simulink model "Robust_joint_Space"  (R2020b)
settings: Solver=VariableStepAuto  StartTime=0.0  StopTime=10  RelTol=1e-3
(part 7 of 7)

== matlab function Robust_joint_Space/robust inverse dynamic controller/M_hat_prod ==
  data: m input; Mhat output; theta input
function Mhat = Find_M(m,theta)

m1 = m(1);
m2 = m(2);
m3 = m(3);
m4 = m(4);
m5 = m(5);
m6 = m(6);

t1 = theta(1);
t2 = theta(2);
t3 = theta(3);
t4 = theta(4);
t5 = theta(5);
t6 = theta(6);

L1=0.1025;
L2=0.408;
L3=0.376;
L4=0.1025; 
L5=0.1025;

Mhat =[(78961*m2)/4 + (411889*m3)/4 + (694641*m4)/4 + (1431307*m5)/8 + (1431307*m6)/8 + (61463515545781917*cos(2*t2))/1152921504606846976 - 83232*m3*cos(2*t2) - 83232*m4*cos(2*t2) - 83232*m5*cos(2*t2) - 83232*m6*cos(2*t2) - (42025*m5*cos(2*t2 + 2*t3 + 2*t4))/8 - (42025*m6*cos(2*t2 + 2*t3 + 2*t4))/8 - 281*L1*m3 - 281*L1*m4 - (205*L4*m5)/2 - 70688*m4*cos(2*t2 + 2*t3) - 70688*m5*cos(2*t2 + 2*t3) - 70688*m6*cos(2*t2 + 2*t3) - 41820*m5*cos(2*t2 + t3 + t4) - 41820*m6*cos(2*t2 + t3 + t4) + 41820*m5*cos(t3 + t4) + 41820*m6*cos(t3 + t4) + L1^2*m3 + (L2^2*m2)/8 + L1^2*m4 + (3*L3^2*m5)/16 + (L4^2*m5)/2 + 153408*m4*cos(t3) + 153408*m5*cos(t3) + 38540*m5*cos(t4) + 153408*m6*cos(t3) + 38540*m6*cos(t4) - 38540*m5*cos(2*t2 + 2*t3 + t4) - 38540*m6*cos(2*t2 + 2*t3 + t4) - 153408*m4*cos(2*t2 + t3) - 153408*m5*cos(2*t2 + t3) - 153408*m6*cos(2*t2 + t3) + 102*L3*m5*cos(2*t2 + t3 + t4 + t5) + 94*L3*m5*cos(t4 - t5) - (205*L3*m5*cos(2*t2 + 2*t3 + 2*t4 - t5))/8 - 102*L3*m5*cos(t3 + t4 + t5) + (205*L4*m5*cos(2*t2 + 2*t3 + 2*t4))/2 - 102*L3*m5*cos(2*t2 + t3 + t4 - t5) + 94*L3*m5*cos(2*t2 + 2*t3 + t4 + t5) - (L3^2*m5*cos(2*t2 + 2*t3 + 2*t4 - 2*t5))/32 - (L3^2*m5*cos(2*t2 + 2*t3 + 2*t4 + 2*t5))/32 + 408*L4*m5*cos(2*t2 + t3 + t4) + 102*L3*m5*cos(t3 + t4 - t5) - (L2^2*m2*cos(2*t2))/8 + (L3^2*m5*cos(2*t5))/16 + (L3^2*m5*cos(2*t2 + 2*t3 + 2*t4))/16 - (L4^2*m5*cos(2*t2 + 2*t3 + 2*t4))/2 - 408*L4*m5*cos(t3 + t4) - 94*L3*m5*cos(t4 + t5) - 94*L3*m5*cos(2*t2 + 2*t3 + t4 - t5) + (205*L3*m5*cos(2*t2 + 2*t3 + 2*t4 + t5))/8 + (281*L3*m5*cos(t5))/2 - 376*L4*m5*cos(t4) + 376*L4*m5*cos(2*t2 + 2*t3 + t4) - (L3*L4*m5*cos(2*t2 + 2*t3 + 2*t4 + t5))/4 + (L3*L4*m5*cos(2*t2 + 2*t3 + 2*t4 - t5))/4 + 204764811175443545/1152921504606846976,                                                                                                                                                                      (61463515545781917*cos(t1 + 2*t2))/2305843009213693952 - (61463515545781917*cos(t1 - 2*t2))/2305843009213693952 - 52828*m4*cos(t2 + t3) - 52828*m5*cos(t2 + t3) - 52828*m6*cos(t2 + t3) - 57324*m3*cos(t2) - 57324*m4*cos(t2) - 57324*m5*cos(t2) - 57324*m6*cos(t2) - (57605*m5*cos(t2 + t3 + t4))/4 - (57605*m6*cos(t2 + t3 + t4))/4 - (243*L3*m5*cos(t2 + t3 + t4 - t5))/4 - (281*L2*m2*cos(t1 - t2))/8 - 102*L3*m5*cos(t2 - t5) - 94*L3*m5*cos(t2 + t3 + t5) + (281*L4*m5*cos(t2 + t3 + t4))/2 - (L3^2*m5*cos(t2 + t3 + t4 - 2*t5))/16 + (L3^2*m5*cos(t2 + t3 + t4 + 2*t5))/16 - (L2^2*m2*cos(t1 - 2*t2))/16 + (L2^2*m2*cos(t1 + 2*t2))/16 - 94*L3*m5*cos(t2 + t3 - t5) + (19*L3*m5*cos(t2 + t3 + t4 + t5))/2 - (281*L2*m2*cos(t1 + t2))/8 + 376*L1*m4*cos(t2 + t3) - 102*L3*m5*cos(t2 + t5) + 408*L1*m3*cos(t2) + 408*L1*m4*cos(t2) + (L3*L4*m5*cos(t2 + t3 + t4 - t5))/4 + (L3*L4*m5*cos(t2 + t3 + t4 + t5))/4,                                                                                                                                                                                                                                                                                                      (1690603261718859*cos(t1 - 2*t2))/2305843009213693952 - (1690603261718859*cos(t1 + 2*t2))/2305843009213693952 - 52828*m4*cos(t2 + t3) - 52828*m5*cos(t2 + t3) - 52828*m6*cos(t2 + t3) - (57605*m5*cos(t2 + t3 + t4))/4 - (57605*m6*cos(t2 + t3 + t4))/4 - (243*L3*m5*cos(t2 + t3 + t4 - t5))/4 - 94*L3*m5*cos(t2 + t3 + t5) + (281*L4*m5*cos(t2 + t3 + t4))/2 - (L3^2*m5*cos(t2 + t3 + t4 - 2*t5))/16 + (L3^2*m5*cos(t2 + t3 + t4 + 2*t5))/16 - 94*L3*m5*cos(t2 + t3 - t5) + (19*L3*m5*cos(t2 + t3 + t4 + t5))/2 + 376*L1*m4*cos(t2 + t3) + (L3*L4*m5*cos(t2 + t3 + t4 - t5))/4 + (L3*L4*m5*cos(t2 + t3 + t4 + t5))/4,                                                                                                                                                                                                                                                                                                                                                                                                                 (1690603261718859*cos(t1 - 2*t2))/2305843009213693952 - (1690603261718859*cos(t1 + 2*t2))/2305843009213693952 - (57605*m5*cos(t2 + t3 + t4))/4 - (57605*m6*cos(t2 + t3 + t4))/4 - (243*L3*m5*cos(t2 + t3 + t4 - t5))/4 + (281*L4*m5*cos(t2 + t3 + t4))/2 - (L3^2*m5*cos(t2 + t3 + t4 - 2*t5))/16 + (L3^2*m5*cos(t2 + t3 + t4 + 2*t5))/16 + (19*L3*m5*cos(t2 + t3 + t4 + t5))/2 + (L3*L4*m5*cos(t2 + t3 + t4 - t5))/4 + (L3*L4*m5*cos(t2 + t3 + t4 + t5))/4,                                                                                                                                                                                                                                                                                                                                                                                                                                                                                                                                                                                                                                             (1690603261718859*cos(t2 + t3 + t4))/1152921504606846976 - (1690603261718859*cos(t1 + t2 - t3 - t4))/4611686018427387904 + (1690603261718859*cos(3*t2 - t1 + t3 + t4))/4611686018427387904 - (1690603261718859*cos(t3 - t2 + t4))/2305843009213693952 - (1690603261718859*cos(3*t2 + t3 + t4))/2305843009213693952 - (1690603261718859*cos(t1 - t2 + t3 + t4))/4611686018427387904 + (1690603261718859*cos(t1 + 3*t2 + t3 + t4))/4611686018427387904 + (19*L3*m5*cos(t2 + t3 + t4 - t5))/2 - 102*L3*m5*cos(t2 - t5) + 94*L3*m5*cos(t2 + t3 + t5) - 94*L3*m5*cos(t2 + t3 - t5) + (L3^2*m5*cos(t2 + t3 + t4))/4 + (243*L3*m5*cos(t2 + t3 + t4 + t5))/4 + 102*L3*m5*cos(t2 + t5) + (L3*L4*m5*cos(t2 + t3 + t4 - t5))/4 - (L3*L4*m5*cos(t2 + t3 + t4 + t5))/4,                                                                                                                                                                                                                                                                                                                                                                                                                                                                                                                                                                                                                                                                                                                                                                                                                                                                                                                                                                                                                                                                                                                                                                               0
                                                                                                                                                                                                                                                                                                                                                                                                                                                                                                                                                                                                                                                                                                                                                                                                                                                          (61463515545781917*cos(t1 + 2*t2))/2305843009213693952 - (61463515545781917*cos(t1 - 2*t2))/2305843009213693952 - 52828*m4*cos(t2 + t3) - 52828*m5*cos(t2 + t3) - 52828*m6*cos(t2 + t3) - 57324*m3*cos(t2) - 57324*m4*cos(t2) - 57324*m5*cos(t2) - 57324*m6*cos(t2) - (57605*m5*cos(t2 + t3 + t4))/4 - (57605*m6*cos(t2 + t3 + t4))/4 - (243*L3*m5*cos(t2 + t3 + t4 - t5))/4 - (281*L2*m2*cos(t1 - t2))/8 - 102*L3*m5*cos(t2 - t5) - 94*L3*m5*cos(t2 + t3 + t5) + (281*L4*m5*cos(t2 + t3 + t4))/2 - (L3^2*m5*cos(t2 + t3 + t4 - 2*t5))/16 + (L3^2*m5*cos(t2 + t3 + t4 + 2*t5))/16 - (L2^2*m2*cos(t1 - 2*t2))/16 + (L2^2*m2*cos(t1 + 2*t2))/16 - 94*L3*m5*cos(t2 + t3 - t5) + (19*L3*m5*cos(t2 + t3 + t4 + t5))/2 - (281*L2*m2*cos(t1 + t2))/8 + 376*L1*m4*cos(t2 + t3) - 102*L3*m5*cos(t2 + t5) + 408*L1*m3*cos(t2) + 408*L1*m4*cos(t2) + (L3*L4*m5*cos(t2 + t3 + t4 - t5))/4 + (L3*L4*m5*cos(t2 + t3 + t4 + t5))/4, (78961*m2)/4 + 166464*m3 + 307840*m4 + (1273385*m5)/4 + (1273385*m6)/4 - (78961*m2*cos(t1)^2)/4 - 205*L4*m5 - (482729437821091191*cos(t1)^2)/4611686018427387904 - (61463515545781917*cos(t2)^2)/576460752303423488 + (1690603261718859*cos(t3)^2)/576460752303423488 + (L3^2*m5)/4 + L4^2*m5 + 306816*m4*cos(t3) + 306816*m5*cos(t3) + 77080*m5*cos(t4) + 306816*m6*cos(t3) + 77080*m6*cos(t4) + (61463515545781917*cos(t1)^2*cos(t2)^2)/576460752303423488 - (1690603261718859*cos(t1)^2*cos(t3)^2)/288230376151711744 + 83640*m5*cos(t3)*cos(t4) + 83640*m6*cos(t3)*cos(t4) - 83640*m5*sin(t3)*sin(t4) - 83640*m6*sin(t3)*sin(t4) + (L2^2*m2*cos(t1)^2)/4 + (L2^2*m2*cos(t2)^2)/4 - (L3^2*m5*cos(t5)^2)/4 - 752*L4*m5*cos(t4) - 816*L4*m5*cos(t3)*cos(t4) - (1690603261718859*cos(t1)*cos(t3)*sin(t1)*sin(t3))/288230376151711744 - (L2^2*m2*cos(t1)^2*cos(t2)^2)/4 + 816*L4*m5*sin(t3)*sin(t4) + 376*L3*m5*sin(t4)*sin(t5) - (281*L2*m2*cos(t1)*sin(t1)*sin(t2))/2 + 408*L3*m5*cos(t3)*sin(t4)*sin(t5) + 408*L3*m5*cos(t4)*sin(t3)*sin(t5) + 1045114580761903793/4611686018427387904,                                                                                                                                                                             141376*m4 + (607529*m5)/4 + (607529*m6)/4 + (2216273498288709*cos(2*t1))/9223372036854775808 + (1690603261718859*cos(2*t2))/2305843009213693952 - (1690603261718859*cos(2*t1 - 2*t2))/4611686018427387904 - (1690603261718859*cos(2*t1 + 2*t2))/4611686018427387904 - (1690603261718859*cos(2*t1 - 2*t3))/1152921504606846976 - 205*L4*m5 + 41820*m5*cos(t3 + t4) + 41820*m6*cos(t3 + t4) + (L3^2*m5)/8 + L4^2*m5 + 153408*m4*cos(t3) + 153408*m5*cos(t3) + 77080*m5*cos(t4) + 153408*m6*cos(t3) + 77080*m6*cos(t4) + 188*L3*m5*cos(t4 - t5) - 102*L3*m5*cos(t3 + t4 + t5) + 102*L3*m5*cos(t3 + t4 - t5) - (L3^2*m5*cos(2*t5))/8 - 408*L4*m5*cos(t3 + t4) - 188*L3*m5*cos(t4 + t5) - 752*L4*m5*cos(t4) + 98563285369573207/9223372036854775808,                                                                                                                                                                                                        (42025*m5)/4 + (42025*m6)/4 + (10637310166265011*cos(2*t1))/9223372036854775808 + (1690603261718859*cos(2*t2))/2305843009213693952 - (1690603261718859*cos(2*t1 - 2*t2))/4611686018427387904 - (1690603261718859*cos(2*t1 + 2*t2))/4611686018427387904 - (1690603261718859*cos(2*t1 - 2*t3))/1152921504606846976 - 205*L4*m5 + 41820*m5*cos(t3 + t4) + 41820*m6*cos(t3 + t4) + (L3^2*m5)/8 + L4^2*m5 + 38540*m5*cos(t4) + 38540*m6*cos(t4) + 94*L3*m5*cos(t4 - t5) - 102*L3*m5*cos(t3 + t4 + t5) + 102*L3*m5*cos(t3 + t4 - t5) - (L3^2*m5*cos(2*t5))/8 - 408*L4*m5*cos(t3 + t4) - 94*L3*m5*cos(t4 + t5) - 376*L4*m5*cos(t4) + 90142248701596905/9223372036854775808,                                                                                                                                                                                                                                                                                                                                                                                                                (1690603261718859*cos(2*t1 + t2 - t3 + t4))/2305843009213693952 - (1690603261718859*cos(t1 + t2 - t3 - t4))/4611686018427387904 + (1690603261718859*cos(2*t1 - t2 + t3 + t4))/9223372036854775808 + (1690603261718859*cos(3*t2 - t1 + t3 + t4))/4611686018427387904 - (1690603261718859*cos(t2 - 2*t1 + 3*t3 + t4))/2305843009213693952 - (1690603261718859*cos(3*t2 - 2*t1 + t3 + t4))/9223372036854775808 + (1690603261718859*cos(2*t1 + 3*t2 + t3 + t4))/9223372036854775808 - (1690603261718859*cos(2*t1 + t2 - t3 - t4))/9223372036854775808 + (1690603261718859*cos(t1 - t2 + t3 + t4))/4611686018427387904 + (10637310166265011*cos(t2 - 2*t1 + t3 + t4))/18446744073709551616 - (10637310166265011*cos(2*t1 + t2 + t3 + t4))/18446744073709551616 - (1690603261718859*cos(t1 + 3*t2 + t3 + t4))/4611686018427387904 - 94*L3*m5*cos(t4 - t5) - 102*L3*m5*cos(t3 + t4 + t5) - 102*L3*m5*cos(t3 + t4 - t5) - 94*L3*m5*cos(t4 + t5) - (205*L3*m5*cos(t5))/4 + (L3*L4*m5*cos(t5))/2,                                                                                                                                                                                                                                                                                                                                                                                                                                                                                                                                                                                                                                                                                                   (3874897119389575*cos(t5))/4611686018427387904 + (3874897119389575*cos(t1)^2*cos(t5))/4611686018427387904 - (3874897119389575*cos(t1)*cos(t2)*cos(t3)*cos(t4)*sin(t1)*sin(t5))/4611686018427387904 + (3874897119389575*cos(t1)*cos(t2)*sin(t1)*sin(t3)*sin(t4)*sin(t5))/4611686018427387904 + (3874897119389575*cos(t1)*cos(t3)*sin(t1)*sin(t2)*sin(t4)*sin(t5))/4611686018427387904 + (3874897119389575*cos(t1)*cos(t4)*sin(t1)*sin(t2)*sin(t3)*sin(t5))/4611686018427387904
                                                                                                                                                                                                                                                                                                                                                                                                                                                                                                                                                                                                                                                                                                                                                                                                                                                                                                                                                                                                                                                                                                                                                        (1690603261718859*cos(t1 - 2*t2))/2305843009213693952 - (1690603261718859*cos(t1 + 2*t2))/2305843009213693952 - 52828*m4*cos(t2 + t3) - 52828*m5*cos(t2 + t3) - 52828*m6*cos(t2 + t3) - (57605*m5*cos(t2 + t3 + t4))/4 - (57605*m6*cos(t2 + t3 + t4))/4 - (243*L3*m5*cos(t2 + t3 + t4 - t5))/4 - 94*L3*m5*cos(t2 + t3 + t5) + (281*L4*m5*cos(t2 + t3 + t4))/2 - (L3^2*m5*cos(t2 + t3 + t4 - 2*t5))/16 + (L3^2*m5*cos(t2 + t3 + t4 + 2*t5))/16 - 94*L3*m5*cos(t2 + t3 - t5) + (19*L3*m5*cos(t2 + t3 + t4 + t5))/2 + 376*L1*m4*cos(t2 + t3) + (L3*L4*m5*cos(t2 + t3 + t4 - t5))/4 + (L3*L4*m5*cos(t2 + t3 + t4 + t5))/4,                                                                                                                                                                                                                                                                                                                                           141376*m4 + (607529*m5)/4 + (607529*m6)/4 + (2216273498288709*cos(2*t1))/9223372036854775808 + (1690603261718859*cos(2*t2))/2305843009213693952 - (1690603261718859*cos(2*t1 - 2*t2))/4611686018427387904 - (1690603261718859*cos(2*t1 + 2*t2))/4611686018427387904 - (1690603261718859*cos(2*t1 - 2*t3))/1152921504606846976 - 205*L4*m5 + 41820*m5*cos(t3 + t4) + 41820*m6*cos(t3 + t4) + (L3^2*m5)/8 + L4^2*m5 + 153408*m4*cos(t3) + 153408*m5*cos(t3) + 77080*m5*cos(t4) + 153408*m6*cos(t3) + 77080*m6*cos(t4) + 188*L3*m5*cos(t4 - t5) - 102*L3*m5*cos(t3 + t4 + t5) + 102*L3*m5*cos(t3 + t4 - t5) - (L3^2*m5*cos(2*t5))/8 - 408*L4*m5*cos(t3 + t4) - 188*L3*m5*cos(t4 + t5) - 752*L4*m5*cos(t4) + 98563285369573207/9223372036854775808,                                                                                                                                                                                                                                                                                                                                141376*m4 + (607529*m5)/4 + (607529*m6)/4 - 205*L4*m5 + (22503512638915017*cos(t1)^2)/4611686018427387904 + (1690603261718859*cos(t2)^2)/576460752303423488 + (1690603261718859*cos(t3)^2)/576460752303423488 + (L3^2*m5)/4 + L4^2*m5 + 77080*m5*cos(t4) + 77080*m6*cos(t4) - (1690603261718859*cos(t1)^2*cos(t2)^2)/576460752303423488 - (1690603261718859*cos(t1)^2*cos(t3)^2)/288230376151711744 - (L3^2*m5*cos(t5)^2)/4 - 752*L4*m5*cos(t4) - (1690603261718859*cos(t1)*cos(t3)*sin(t1)*sin(t3))/288230376151711744 + 376*L3*m5*sin(t4)*sin(t5) + 34648679841891377/4611686018427387904,                                                                                                                                                                                                                                                                                              (42025*m5)/4 + (42025*m6)/4 - 205*L4*m5 + (30924549306891319*cos(t1)^2)/4611686018427387904 + (1690603261718859*cos(t2)^2)/576460752303423488 + (1690603261718859*cos(t3)^2)/576460752303423488 + (L3^2*m5)/4 + L4^2*m5 + 38540*m5*cos(t4) + 38540*m6*cos(t4) - (1690603261718859*cos(t1)^2*cos(t2)^2)/576460752303423488 - (1690603261718859*cos(t1)^2*cos(t3)^2)/288230376151711744 - (L3^2*m5*cos(t5)^2)/4 - 376*L4*m5*cos(t4) - (1690603261718859*cos(t1)*cos(t3)*sin(t1)*sin(t3))/288230376151711744 + 188*L3*m5*sin(t4)*sin(t5) + 26227643173915075/4611686018427387904,                                                                                                                                                                                                                                                                                                                                                                                                                                                                            (1690603261718859*cos(2*t1 + t2 - t3 + t4))/2305843009213693952 - (1690603261718859*cos(t1 + t2 - t3 - t4))/4611686018427387904 + (1690603261718859*cos(2*t1 - t2 + t3 + t4))/9223372036854775808 + (1690603261718859*cos(3*t2 - t1 + t3 + t4))/4611686018427387904 - (1690603261718859*cos(t2 - 2*t1 + 3*t3 + t4))/2305843009213693952 - (1690603261718859*cos(3*t2 - 2*t1 + t3 + t4))/9223372036854775808 + (1690603261718859*cos(2*t1 + 3*t2 + t3 + t4))/9223372036854775808 - (1690603261718859*cos(2*t1 + t2 - t3 - t4))/9223372036854775808 + (1690603261718859*cos(t1 - t2 + t3 + t4))/4611686018427387904 + (10637310166265011*cos(t2 - 2*t1 + t3 + t4))/18446744073709551616 - (10637310166265011*cos(2*t1 + t2 + t3 + t4))/18446744073709551616 - (1690603261718859*cos(t1 + 3*t2 + t3 + t4))/4611686018427387904 - 94*L3*m5*cos(t4 - t5) - 94*L3*m5*cos(t4 + t5) - (205*L3*m5*cos(t5))/4 + (L3*L4*m5*cos(t5))/2,                                                                                                                                                                                                                                                                                                                                                                                                                                                                                                                                                                                                                                                                                                   (3874897119389575*cos(t5))/4611686018427387904 + (3874897119389575*cos(t1)^2*cos(t5))/4611686018427387904 - (3874897119389575*cos(t1)*cos(t2)*cos(t3)*cos(t4)*sin(t1)*sin(t5))/4611686018427387904 + (3874897119389575*cos(t1)*cos(t2)*sin(t1)*sin(t3)*sin(t4)*sin(t5))/4611686018427387904 + (3874897119389575*cos(t1)*cos(t3)*sin(t1)*sin(t2)*sin(t4)*sin(t5))/4611686018427387904 + (3874897119389575*cos(t1)*cos(t4)*sin(t1)*sin(t2)*sin(t3)*sin(t5))/4611686018427387904
                                                                                                                                                                                                                                                                                                                                                                                                                                                                                                                                                                                                                                                                                                                                                                                                                                                                                                                                                                                                                                                                                                                                                                                                                                                                                                                   (1690603261718859*cos(t1 - 2*t2))/2305843009213693952 - (1690603261718859*cos(t1 + 2*t2))/2305843009213693952 - (57605*m5*cos(t2 + t3 + t4))/4 - (57605*m6*cos(t2 + t3 + t4))/4 - (243*L3*m5*cos(t2 + t3 + t4 - t5))/4 + (281*L4*m5*cos(t2 + t3 + t4))/2 - (L3^2*m5*cos(t2 + t3 + t4 - 2*t5))/16 + (L3^2*m5*cos(t2 + t3 + t4 + 2*t5))/16 + (19*L3*m5*cos(t2 + t3 + t4 + t5))/2 + (L3*L4*m5*cos(t2 + t3 + t4 - t5))/4 + (L3*L4*m5*cos(t2 + t3 + t4 + t5))/4,                                                                                                                                                                                                                                                                                                                                                                                                                      (42025*m5)/4 + (42025*m6)/4 + (10637310166265011*cos(2*t1))/9223372036854775808 + (1690603261718859*cos(2*t2))/2305843009213693952 - (1690603261718859*cos(2*t1 - 2*t2))/4611686018427387904 - (1690603261718859*cos(2*t1 + 2*t2))/4611686018427387904 - (1690603261718859*cos(2*t1 - 2*t3))/1152921504606846976 - 205*L4*m5 + 41820*m5*cos(t3 + t4) + 41820*m6*cos(t3 + t4) + (L3^2*m5)/8 + L4^2*m5 + 38540*m5*cos(t4) + 38540*m6*cos(t4) + 94*L3*m5*cos(t4 - t5) - 102*L3*m5*cos(t3 + t4 + t5) + 102*L3*m5*cos(t3 + t4 - t5) - (L3^2*m5*cos(2*t5))/8 - 408*L4*m5*cos(t3 + t4) - 94*L3*m5*cos(t4 + t5) - 376*L4*m5*cos(t4) + 90142248701596905/9223372036854775808,                                                                                                                                                                                                                                                                                                                                              (42025*m5)/4 + (42025*m6)/4 - 205*L4*m5 + (30924549306891319*cos(t1)^2)/4611686018427387904 + (1690603261718859*cos(t2)^2)/576460752303423488 + (1690603261718859*cos(t3)^2)/576460752303423488 + (L3^2*m5)/4 + L4^2*m5 + 38540*m5*cos(t4) + 38540*m6*cos(t4) - (1690603261718859*cos(t1)^2*cos(t2)^2)/576460752303423488 - (1690603261718859*cos(t1)^2*cos(t3)^2)/288230376151711744 - (L3^2*m5*cos(t5)^2)/4 - 376*L4*m5*cos(t4) - (1690603261718859*cos(t1)*cos(t3)*sin(t1)*sin(t3))/288230376151711744 + 188*L3*m5*sin(t4)*sin(t5) + 26227643173915075/4611686018427387904,                                                                                                                                                                                                                                                                                                                                                                                                                                              (42025*m5)/4 + (42025*m6)/4 + (10637310166265011*cos(2*t1))/9223372036854775808 + (1690603261718859*cos(2*t2))/2305843009213693952 - 205*L4*m5 + (L3^2*m5)/8 + L4^2*m5 - (1690603261718859*cos(2*t1)*cos(2*t2))/2305843009213693952 - (1690603261718859*cos(2*t1)*cos(2*t3))/1152921504606846976 - (1690603261718859*sin(2*t1)*sin(2*t3))/1152921504606846976 - (L3^2*m5*cos(2*t5))/8 + 90142248701596905/9223372036854775808,                                                                                                                                                                                                                                                                                                                                                                                                                                                                                                                            (1690603261718859*cos(2*t1 + t2 - t3 + t4))/2305843009213693952 - (1690603261718859*cos(t1 + t2 - t3 - t4))/4611686018427387904 + (1690603261718859*cos(2*t1 - t2 + t3 + t4))/9223372036854775808 + (1690603261718859*cos(3*t2 - t1 + t3 + t4))/4611686018427387904 - (1690603261718859*cos(t2 - 2*t1 + 3*t3 + t4))/2305843009213693952 - (1690603261718859*cos(3*t2 - 2*t1 + t3 + t4))/9223372036854775808 + (1690603261718859*cos(2*t1 + 3*t2 + t3 + t4))/9223372036854775808 - (1690603261718859*cos(2*t1 + t2 - t3 - t4))/9223372036854775808 + (1690603261718859*cos(t1 - t2 + t3 + t4))/4611686018427387904 + (10637310166265011*cos(t2 - 2*t1 + t3 + t4))/18446744073709551616 - (10637310166265011*cos(2*t1 + t2 + t3 + t4))/18446744073709551616 - (1690603261718859*cos(t1 + 3*t2 + t3 + t4))/4611686018427387904 - (205*L3*m5*cos(t5))/4 + (L3*L4*m5*cos(t5))/2,                                                                                                                                                                                                                                                                                                                                                                                                                                                                                                                                                                                                                                                                                                   (3874897119389575*cos(t5))/4611686018427387904 + (3874897119389575*cos(t1)^2*cos(t5))/4611686018427387904 - (3874897119389575*cos(t1)*cos(t2)*cos(t3)*cos(t4)*sin(t1)*sin(t5))/4611686018427387904 + (3874897119389575*cos(t1)*cos(t2)*sin(t1)*sin(t3)*sin(t4)*sin(t5))/4611686018427387904 + (3874897119389575*cos(t1)*cos(t3)*sin(t1)*sin(t2)*sin(t4)*sin(t5))/4611686018427387904 + (3874897119389575*cos(t1)*cos(t4)*sin(t1)*sin(t2)*sin(t3)*sin(t5))/4611686018427387904
                                                                                                                                                                                                                                                                                                                                                                                                                                                                                                                                                                                                                                                                                                                                                                                                                                                                                                                                                                                                                    (1690603261718859*cos(t2 + t3 + t4))/1152921504606846976 - (1690603261718859*cos(t1 + t2 - t3 - t4))/4611686018427387904 + (1690603261718859*cos(3*t2 - t1 + t3 + t4))/4611686018427387904 - (1690603261718859*cos(t3 - t2 + t4))/2305843009213693952 - (1690603261718859*cos(3*t2 + t3 + t4))/2305843009213693952 - (1690603261718859*cos(t1 - t2 + t3 + t4))/4611686018427387904 + (1690603261718859*cos(t1 + 3*t2 + t3 + t4))/4611686018427387904 + (19*L3*m5*cos(t2 + t3 + t4 - t5))/2 - 102*L3*m5*cos(t2 - t5) + 94*L3*m5*cos(t2 + t3 + t5) - 94*L3*m5*cos(t2 + t3 - t5) + (L3^2*m5*cos(t2 + t3 + t4))/4 + (243*L3*m5*cos(t2 + t3 + t4 + t5))/4 + 102*L3*m5*cos(t2 + t5) + (L3*L4*m5*cos(t2 + t3 + t4 - t5))/4 - (L3*L4*m5*cos(t2 + t3 + t4 + t5))/4,                                                                                                   (1690603261718859*cos(2*t1 + t2 - t3 + t4))/2305843009213693952 - (1690603261718859*cos(t1 + t2 - t3 - t4))/4611686018427387904 + (1690603261718859*cos(2*t1 - t2 + t3 + t4))/9223372036854775808 + (1690603261718859*cos(3*t2 - t1 + t3 + t4))/4611686018427387904 - (1690603261718859*cos(t2 - 2*t1 + 3*t3 + t4))/2305843009213693952 - (1690603261718859*cos(3*t2 - 2*t1 + t3 + t4))/9223372036854775808 + (1690603261718859*cos(2*t1 + 3*t2 + t3 + t4))/9223372036854775808 - (1690603261718859*cos(2*t1 + t2 - t3 - t4))/9223372036854775808 + (1690603261718859*cos(t1 - t2 + t3 + t4))/4611686018427387904 + (10637310166265011*cos(t2 - 2*t1 + t3 + t4))/18446744073709551616 - (10637310166265011*cos(2*t1 + t2 + t3 + t4))/18446744073709551616 - (1690603261718859*cos(t1 + 3*t2 + t3 + t4))/4611686018427387904 - 94*L3*m5*cos(t4 - t5) - 102*L3*m5*cos(t3 + t4 + t5) - 102*L3*m5*cos(t3 + t4 - t5) - 94*L3*m5*cos(t4 + t5) - (205*L3*m5*cos(t5))/4 + (L3*L4*m5*cos(t5))/2, (1690603261718859*cos(2*t1 + t2 - t3 + t4))/2305843009213693952 - (1690603261718859*cos(t1 + t2 - t3 - t4))/4611686018427387904 + (1690603261718859*cos(2*t1 - t2 + t3 + t4))/9223372036854775808 + (1690603261718859*cos(3*t2 - t1 + t3 + t4))/4611686018427387904 - (1690603261718859*cos(t2 - 2*t1 + 3*t3 + t4))/2305843009213693952 - (1690603261718859*cos(3*t2 - 2*t1 + t3 + t4))/9223372036854775808 + (1690603261718859*cos(2*t1 + 3*t2 + t3 + t4))/9223372036854775808 - (1690603261718859*cos(2*t1 + t2 - t3 - t4))/9223372036854775808 + (1690603261718859*cos(t1 - t2 + t3 + t4))/4611686018427387904 + (10637310166265011*cos(t2 - 2*t1 + t3 + t4))/18446744073709551616 - (10637310166265011*cos(2*t1 + t2 + t3 + t4))/18446744073709551616 - (1690603261718859*cos(t1 + 3*t2 + t3 + t4))/4611686018427387904 - 94*L3*m5*cos(t4 - t5) - 94*L3*m5*cos(t4 + t5) - (205*L3*m5*cos(t5))/4 + (L3*L4*m5*cos(t5))/2, (1690603261718859*cos(2*t1 + t2 - t3 + t4))/2305843009213693952 - (1690603261718859*cos(t1 + t2 - t3 - t4))/4611686018427387904 + (1690603261718859*cos(2*t1 - t2 + t3 + t4))/9223372036854775808 + (1690603261718859*cos(3*t2 - t1 + t3 + t4))/4611686018427387904 - (1690603261718859*cos(t2 - 2*t1 + 3*t3 + t4))/2305843009213693952 - (1690603261718859*cos(3*t2 - 2*t1 + t3 + t4))/9223372036854775808 + (1690603261718859*cos(2*t1 + 3*t2 + t3 + t4))/9223372036854775808 - (1690603261718859*cos(2*t1 + t2 - t3 - t4))/9223372036854775808 + (1690603261718859*cos(t1 - t2 + t3 + t4))/4611686018427387904 + (10637310166265011*cos(t2 - 2*t1 + t3 + t4))/18446744073709551616 - (10637310166265011*cos(2*t1 + t2 + t3 + t4))/18446744073709551616 - (1690603261718859*cos(t1 + 3*t2 + t3 + t4))/4611686018427387904 - (205*L3*m5*cos(t5))/4 + (L3*L4*m5*cos(t5))/2, (m5*L3^2)/4 + (10637310166265011*cos(2*t2 - 2*t1 + 2*t3 + 2*t4))/36893488147419103232 + (10637310166265011*cos(2*t1 + 2*t2 + 2*t3 + 2*t4))/36893488147419103232 + (1690603261718859*cos(4*t2 - t1 + 2*t3 + 2*t4))/4611686018427387904 - (1690603261718859*cos(2*t2 - 2*t1 + 4*t3 + 2*t4))/4611686018427387904 - (1690603261718859*cos(4*t2 - 2*t1 + 2*t3 + 2*t4))/18446744073709551616 - (1690603261718859*cos(2*t1 + 4*t2 + 2*t3 + 2*t4))/18446744073709551616 - (10637310166265011*cos(2*t1))/18446744073709551616 - (1690603261718859*cos(2*t2))/4611686018427387904 - (1690603261718859*cos(2*t3 - t1 + 2*t4))/4611686018427387904 - (1690603261718859*cos(2*t1 + 2*t2 + 2*t4))/4611686018427387904 - (1690603261718859*cos(2*t3 - 2*t1 + 2*t4))/18446744073709551616 - (1690603261718859*cos(2*t1 + 2*t3 + 2*t4))/18446744073709551616 - (31911930498795033*cos(2*t2 + 2*t3 + 2*t4))/18446744073709551616 - (5071809785156577*cos(4*t2 + 2*t3 + 2*t4))/9223372036854775808 + (1690603261718859*cos(2*t1 - 2*t2))/9223372036854775808 + (1690603261718859*cos(2*t1 + 2*t2))/9223372036854775808 + (1690603261718859*cos(2*t1 - 2*t3))/2305843009213693952 - (5071809785156577*cos(2*t3 + 2*t4))/9223372036854775808 + (1690603261718859*cos(t1 + 4*t2 + 2*t3 + 2*t4))/4611686018427387904 - (1690603261718859*cos(t1 + 2*t3 + 2*t4))/4611686018427387904 + 58961582686296777/18446744073709551616,                                                                                                                           (11624691358168725*sin(2*t2)*sin(2*t3)*sin(2*t4)*sin(t5))/18446744073709551616 - (11624691358168725*cos(2*t2)*cos(2*t3)*sin(2*t4)*sin(t5))/18446744073709551616 - (11624691358168725*cos(2*t2)*cos(2*t4)*sin(2*t3)*sin(t5))/18446744073709551616 - (11624691358168725*cos(2*t3)*cos(2*t4)*sin(2*t2)*sin(t5))/18446744073709551616 + (3874897119389575*sin(2*t1)*cos(t2)*cos(t3)*cos(t5)*sin(t4))/9223372036854775808 + (3874897119389575*sin(2*t1)*cos(t2)*cos(t4)*cos(t5)*sin(t3))/9223372036854775808 + (3874897119389575*sin(2*t1)*cos(t3)*cos(t4)*cos(t5)*sin(t2))/9223372036854775808 + (3874897119389575*cos(2*t1)*cos(2*t2)*cos(2*t3)*sin(2*t4)*sin(t5))/18446744073709551616 + (3874897119389575*cos(2*t1)*cos(2*t2)*cos(2*t4)*sin(2*t3)*sin(t5))/18446744073709551616 + (3874897119389575*cos(2*t1)*cos(2*t3)*cos(2*t4)*sin(2*t2)*sin(t5))/18446744073709551616 - (3874897119389575*sin(2*t1)*cos(t5)*sin(t2)*sin(t3)*sin(t4))/9223372036854775808 - (3874897119389575*cos(2*t1)*sin(2*t2)*sin(2*t3)*sin(2*t4)*sin(t5))/18446744073709551616
                                                                                                                                                                                                                                                                                                                                                                                                                                                                                                                                                                                                                                                                                                                                                                                                                                                                                                                                                                                                                                                                                                                                                                                                                                                                                                                                                                                                                                                                                                                                                                                                                                                                                                                                                                            0,                                                                                                                                                                                                                                                                                                                                                                                                                                                                                                                                                                                                            (3874897119389575*cos(t5))/4611686018427387904 + (3874897119389575*cos(t1)^2*cos(t5))/4611686018427387904 - (3874897119389575*cos(t1)*cos(t2)*cos(t3)*cos(t4)*sin(t1)*sin(t5))/4611686018427387904 + (3874897119389575*cos(t1)*cos(t2)*sin(t1)*sin(t3)*sin(t4)*sin(t5))/4611686018427387904 + (3874897119389575*cos(t1)*cos(t3)*sin(t1)*sin(t2)*sin(t4)*sin(t5))/4611686018427387904 + (3874897119389575*cos(t1)*cos(t4)*sin(t1)*sin(t2)*sin(t3)*sin(t5))/4611686018427387904,                                                                                                                                                                                                                                                                                                                                                                                                                                              (3874897119389575*cos(t5))/4611686018427387904 + (3874897119389575*cos(t1)^2*cos(t5))/4611686018427387904 - (3874897119389575*cos(t1)*cos(t2)*cos(t3)*cos(t4)*sin(t1)*sin(t5))/4611686018427387904 + (3874897119389575*cos(t1)*cos(t2)*sin(t1)*sin(t3)*sin(t4)*sin(t5))/4611686018427387904 + (3874897119389575*cos(t1)*cos(t3)*sin(t1)*sin(t2)*sin(t4)*sin(t5))/4611686018427387904 + (3874897119389575*cos(t1)*cos(t4)*sin(t1)*sin(t2)*sin(t3)*sin(t5))/4611686018427387904,                                                                                                                                                                                                                                                                                                                                                                                              (3874897119389575*cos(t5))/4611686018427387904 + (3874897119389575*cos(t1)^2*cos(t5))/4611686018427387904 - (3874897119389575*cos(t1)*cos(t2)*cos(t3)*cos(t4)*sin(t1)*sin(t5))/4611686018427387904 + (3874897119389575*cos(t1)*cos(t2)*sin(t1)*sin(t3)*sin(t4)*sin(t5))/4611686018427387904 + (3874897119389575*cos(t1)*cos(t3)*sin(t1)*sin(t2)*sin(t4)*sin(t5))/4611686018427387904 + (3874897119389575*cos(t1)*cos(t4)*sin(t1)*sin(t2)*sin(t3)*sin(t5))/4611686018427387904,                                                                                                                                                                                                                                                                                                                                                 (11624691358168725*sin(2*t2)*sin(2*t3)*sin(2*t4)*sin(t5))/18446744073709551616 - (11624691358168725*cos(2*t2)*cos(2*t3)*sin(2*t4)*sin(t5))/18446744073709551616 - (11624691358168725*cos(2*t2)*cos(2*t4)*sin(2*t3)*sin(t5))/18446744073709551616 - (11624691358168725*cos(2*t3)*cos(2*t4)*sin(2*t2)*sin(t5))/18446744073709551616 + (3874897119389575*sin(2*t1)*cos(t2)*cos(t3)*cos(t5)*sin(t4))/9223372036854775808 + (3874897119389575*sin(2*t1)*cos(t2)*cos(t4)*cos(t5)*sin(t3))/9223372036854775808 + (3874897119389575*sin(2*t1)*cos(t3)*cos(t4)*cos(t5)*sin(t2))/9223372036854775808 + (3874897119389575*cos(2*t1)*cos(2*t2)*cos(2*t3)*sin(2*t4)*sin(t5))/18446744073709551616 + (3874897119389575*cos(2*t1)*cos(2*t2)*cos(2*t4)*sin(2*t3)*sin(t5))/18446744073709551616 + (3874897119389575*cos(2*t1)*cos(2*t3)*cos(2*t4)*sin(2*t2)*sin(t5))/18446744073709551616 - (3874897119389575*sin(2*t1)*cos(t5)*sin(t2)*sin(t3)*sin(t4))/9223372036854775808 - (3874897119389575*cos(2*t1)*sin(2*t2)*sin(2*t3)*sin(2*t4)*sin(t5))/18446744073709551616, ((3874897119389575*cos(t1)*cos(t2)*sin(t3)*sin(t4)*sin(t5))/4611686018427387904 - (3874897119389575*cos(t1)*cos(t2)*cos(t3)*cos(t4)*sin(t5))/4611686018427387904 - (3874897119389575*cos(t5)*sin(t1))/4611686018427387904 + (3874897119389575*cos(t1)*cos(t3)*sin(t2)*sin(t4)*sin(t5))/4611686018427387904 + (3874897119389575*cos(t1)*cos(t4)*sin(t2)*sin(t3)*sin(t5))/4611686018427387904)*(cos(t1)*cos(t2)*sin(t3)*sin(t4)*sin(t5) - cos(t1)*cos(t2)*cos(t3)*cos(t4)*sin(t5) - cos(t5)*sin(t1) + cos(t1)*cos(t3)*sin(t2)*sin(t4)*sin(t5) + cos(t1)*cos(t4)*sin(t2)*sin(t3)*sin(t5)) + ((3874897119389575*cos(t1)*cos(t5))/2305843009213693952 - (3874897119389575*cos(t2)*cos(t3)*cos(t4)*sin(t1)*sin(t5))/2305843009213693952 + (3874897119389575*cos(t2)*sin(t1)*sin(t3)*sin(t4)*sin(t5))/2305843009213693952 + (3874897119389575*cos(t3)*sin(t1)*sin(t2)*sin(t4)*sin(t5))/2305843009213693952 + (3874897119389575*cos(t4)*sin(t1)*sin(t2)*sin(t3)*sin(t5))/2305843009213693952)*(cos(t1)*cos(t5) - cos(t2)*cos(t3)*cos(t4)*sin(t1)*sin(t5) + cos(t2)*sin(t1)*sin(t3)*sin(t4)*sin(t5) + cos(t3)*sin(t1)*sin(t2)*sin(t4)*sin(t5) + cos(t4)*sin(t1)*sin(t2)*sin(t3)*sin(t5))];

== matlab function Robust_joint_Space/robust inverse dynamic controller/a_theta ==
  data: a_theta output; error input; errord input; thetadd_desired input
function a_theta  = innerloop(error,errord,thetadd_desired)

K0= diag([2;2;2;5;5;5]);
K1= diag([0.9;0.9;0.9;0.1;0.1;0.1]);

B=[zeros(6)
   eye(6)];
P = 0.05*eye(12) ;
e=[error
    errord];

% error of robust control;


ro = 10;
lim = B.'*P*e;
if (norm(lim)>0)
    delta_a = -ro*((lim)/norm(lim));
else
    delta_a = zeros(6,1);
end

a_theta = K0*error + K1*errord + thetadd_desired + delta_a;

end
